simulink model "ECEN_5738_Project_sim"  (R2025b)
settings: Solver=VariableStepAuto  StartTime=0.0  StopTime=3  RelTol=1e-3
undefined symbols (not defined in the file): L, m, p1, p2, p3, p4, p5, r, v, x0
settings Model: Creator=jacks  LastModifiedBy=phil

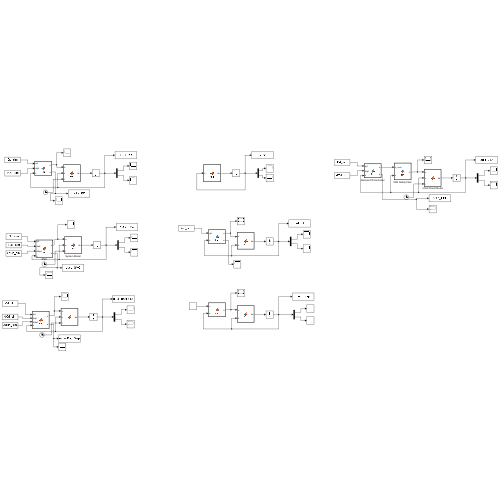
[thumbnail: Simulink's stored preview of the top-level diagram]
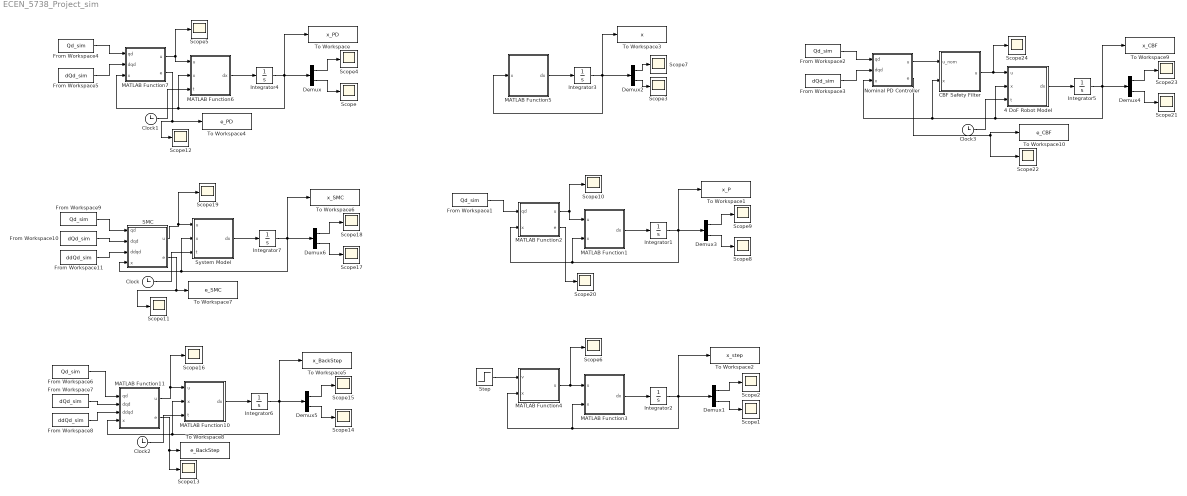
== system ECEN_5738_Project_sim ==
  4 DoF Robot Model : MATLAB Function  TreatAsAtomicUnit=on
  CBF Safety Filter : MATLAB Function  TreatAsAtomicUnit=on
  Clock{,1..3} (4 alike) : Clock
  Demux{,1..6} (7 alike) : Demux  Outputs=2
  From Workspace{1..2,4,6,9} (5 alike) : FromWorkspace  VariableName=Qd_sim
  From Workspace{3,5,7,10} (4 alike) : FromWorkspace  VariableName=dQd_sim
  From Workspace11 : FromWorkspace  VariableName=ddQd_sim
  From Workspace8 : FromWorkspace  VariableName=ddQd_sim
  Integrator{1..7} (7 alike) : Integrator  InitialCondition=x0
  MATLAB Function1 : MATLAB Function  TreatAsAtomicUnit=on
  MATLAB Function10 : MATLAB Function  TreatAsAtomicUnit=on
  MATLAB Function11 : MATLAB Function  TreatAsAtomicUnit=on
  MATLAB Function2 : MATLAB Function  TreatAsAtomicUnit=on
  MATLAB Function3 : MATLAB Function  TreatAsAtomicUnit=on
  MATLAB Function4 : MATLAB Function  TreatAsAtomicUnit=on
  MATLAB Function5 : MATLAB Function  TreatAsAtomicUnit=on
  MATLAB Function6 : MATLAB Function  TreatAsAtomicUnit=on
  MATLAB Function7 : MATLAB Function  TreatAsAtomicUnit=on
  Nominal PD Controller : MATLAB Function  TreatAsAtomicUnit=on
  SMC : MATLAB Function  TreatAsAtomicUnit=on
  Scope{,1..24} (25 alike) : Scope
      Scope settings: ActiveDisplayYMinimum=-1.04346  ActiveDisplayYMaximum=6.65946  DataLoggingVariableName=ScopeData3
      Scope1 settings: ActiveDisplayYMinimum=-0.94669  ActiveDisplayYMaximum=4.37778  DataLoggingVariableName=ScopeData4
      Scope10 settings: ActiveDisplayYMinimum=-1.20532  ActiveDisplayYMaximum=5.7236  DataLoggingVariableName=ScopeData8
      Scope11 settings: ActiveDisplayYMinimum=-0.00123  ActiveDisplayYMaximum=0.00133  DataLoggingVariableName=ScopeData4
      Scope12 settings: ActiveDisplayYMinimum=-0.0028  ActiveDisplayYMaximum=0.00283  DataLoggingVariableName=ScopeData5
      Scope13 settings: ActiveDisplayYMinimum=-0.01077  ActiveDisplayYMaximum=0.01072  DataLoggingVariableName=ScopeData6
      Scope14 settings: ActiveDisplayYMinimum=-1.05117  ActiveDisplayYMaximum=6.70832  DataLoggingVariableName=ScopeData14
      Scope15 settings: ActiveDisplayYMinimum=-2.41084  ActiveDisplayYMaximum=7.25873  DataLoggingVariableName=ScopeData15
      Scope16 settings: ActiveDisplayYMinimum=-4.58136  ActiveDisplayYMaximum=9.58212  DataLoggingVariableName=ScopeData16
      Scope17 settings: ActiveDisplayYMinimum=-1.0429937970844376  ActiveDisplayYMaximum=6.665414521803287
      Scope18 settings: ActiveDisplayYMinimum=-2.4103155124247957  ActiveDisplayYMaximum=7.2502189725166577  DataLoggingVariableName=ScopeData2
      Scope19 settings: ActiveDisplayYMinimum=-4.55981  ActiveDisplayYMaximum=9.43347  DataLoggingVariableName=ScopeData3
      Scope2 settings: ActiveDisplayYMinimum=-2.27232  ActiveDisplayYMaximum=6.12142
      Scope20 settings: ActiveDisplayYMinimum=-0.02858  ActiveDisplayYMaximum=0.02832  DataLoggingVariableName=ScopeData7
      Scope21 settings: ActiveDisplayYMinimum=-0.93914626541497248  ActiveDisplayYMaximum=5.7206527652501826
      Scope22 settings: ActiveDisplayYMinimum=-0.1369  ActiveDisplayYMaximum=0.37912  DataLoggingVariableName=ScopeData2
      Scope23 settings: ActiveDisplayYMinimum=-2.3974052419553082  ActiveDisplayYMaximum=7.1319937805003715  DataLoggingVariableName=ScopeData3
      Scope24 settings: ActiveDisplayYMinimum=-4.5558  ActiveDisplayYMaximum=9.43326  DataLoggingVariableName=ScopeData4
      Scope3 settings: ActiveDisplayYMinimum=-16.16611  ActiveDisplayYMaximum=1.79624
      Scope4 settings: ActiveDisplayYMinimum=-2.41035  ActiveDisplayYMaximum=7.2485  DataLoggingVariableName=ScopeData2
      Scope5 settings: ActiveDisplayYMinimum=-4.55909  ActiveDisplayYMaximum=9.43362  DataLoggingVariableName=ScopeData5
      Scope6 settings: ActiveDisplayYMinimum=-0.16415  ActiveDisplayYMaximum=1.38114  DataLoggingVariableName=ScopeData6
      Scope7 settings: ActiveDisplayYMinimum=-7.05771  ActiveDisplayYMaximum=2.87087  DataLoggingVariableName=ScopeData7
      Scope8 settings: ActiveDisplayYMinimum=-18.16231  ActiveDisplayYMaximum=18.17247  DataLoggingVariableName=ScopeData9
      Scope9 settings: ActiveDisplayYMinimum=-2.41317  ActiveDisplayYMaximum=7.27485  DataLoggingVariableName=ScopeData10
  Step : Step  Time=0  Before=x0(1:4)  After=v  SampleTime=0
  System Model : MATLAB Function  TreatAsAtomicUnit=on
  To Workspace : ToWorkspace  VariableName=x_PD  SaveFormat=Timeseries  SampleTime=-1
  To Workspace1 : ToWorkspace  VariableName=x_P  SaveFormat=Timeseries  SampleTime=-1
  To Workspace10 : ToWorkspace  VariableName=e_CBF  SaveFormat=Timeseries  SampleTime=-1
  To Workspace2 : ToWorkspace  VariableName=x_step  SaveFormat=Timeseries  SampleTime=-1
  To Workspace3 : ToWorkspace  VariableName=x  SaveFormat=Timeseries  SampleTime=-1
  To Workspace4 : ToWorkspace  VariableName=e_PD  SaveFormat=Timeseries  SampleTime=-1
  To Workspace5 : ToWorkspace  VariableName=x_BackStep  SaveFormat=Timeseries  SampleTime=-1
  To Workspace6 : ToWorkspace  VariableName=x_SMC  SaveFormat=Timeseries  SampleTime=-1
  To Workspace7 : ToWorkspace  VariableName=e_SMC  SaveFormat=Timeseries  SampleTime=-1
  To Workspace8 : ToWorkspace  VariableName=e_BackStep  SaveFormat=Timeseries  SampleTime=-1
  To Workspace9 : ToWorkspace  VariableName=x_CBF  SaveFormat=Timeseries  SampleTime=-1
  wires:
  Integrator2/1 -> To Workspace2/1, Demux1/1, MATLAB Function3/2(x), MATLAB Function4/2(x)
  MATLAB Function4/1(u) -> Scope6/1, MATLAB Function3/1(u)
  MATLAB Function3/1(dx) -> Integrator2/1
  Step/1 -> MATLAB Function4/1(v)
  Integrator3/1 -> To Workspace3/1, MATLAB Function5/1(x), Demux2/1
  MATLAB Function5/1(dx) -> Integrator3/1
  From Workspace5/1 -> MATLAB Function7/2(dqd)
  Integrator4/1 -> To Workspace/1, Demux/1, MATLAB Function7/3(x), MATLAB Function6/2(x)
  MATLAB Function6/1(dx) -> Integrator4/1
  MATLAB Function7/1(u) -> MATLAB Function6/1(u), Scope5/1
  From Workspace4/1 -> MATLAB Function7/1(qd)
  Demux/1 -> Scope4/1
  Demux/2 -> Scope/1
  Demux1/2 -> Scope1/1
  Demux1/1 -> Scope2/1
  Demux2/2 -> Scope3/1
  Demux2/1 -> Scope7/1
  Integrator1/1 -> To Workspace1/1, Demux3/1, MATLAB Function2/2(x), MATLAB Function1/2(x)
  MATLAB Function2/1(u) -> MATLAB Function1/1(u), Scope10/1
  From Workspace1/1 -> MATLAB Function2/1(qd)
  MATLAB Function1/1(dx) -> Integrator1/1
  Demux3/1 -> Scope9/1
  Demux3/2 -> Scope8/1
  Integrator6/1 -> To Workspace5/1, Demux5/1, MATLAB Function11/4(x), MATLAB Function10/2(x)
  From Workspace7/1 -> MATLAB Function11/2(dqd)
  MATLAB Function11/1(u) -> Scope16/1, MATLAB Function10/1(u)
  From Workspace6/1 -> MATLAB Function11/1(qd)
  MATLAB Function10/1(dx) -> Integrator6/1
  Demux5/1 -> Scope15/1
  Demux5/2 -> Scope14/1
  From Workspace8/1 -> MATLAB Function11/3(ddqd)
  From Workspace9/1 -> SMC/1(qd)
  Integrator7/1 -> To Workspace6/1, Demux6/1, SMC/4(x), System Model/2(x)
  From Workspace10/1 -> SMC/2(dqd)
  Demux6/2 -> Scope17/1
  System Model/1(dx) -> Integrator7/1
  Demux6/1 -> Scope18/1
  From Workspace11/1 -> SMC/3(ddqd)
  SMC/1(u) -> Scope19/1, System Model/1(u)
  Clock/1 -> System Model/3(t)
  Clock1/1 -> MATLAB Function6/3(t)
  Clock2/1 -> MATLAB Function10/3(t)
  MATLAB Function7/2(e) -> To Workspace4/1, Scope12/1
  SMC/2(e) -> Scope11/1, To Workspace7/1
  MATLAB Function11/2(e) -> Scope13/1, To Workspace8/1
  MATLAB Function2/2(e) -> Scope20/1
  4 DoF Robot Model/1(dx) -> Integrator5/1
  Demux4/1 -> Scope23/1
  Clock3/1 -> 4 DoF Robot Model/3(t)
  Demux4/2 -> Scope21/1
  Nominal PD Controller/2(e) -> To Workspace10/1, Scope22/1
  From Workspace2/1 -> Nominal PD Controller/1(qd)
  From Workspace3/1 -> Nominal PD Controller/2(dqd)
  Integrator5/1 -> To Workspace9/1, Demux4/1, CBF Safety Filter/2(x), Nominal PD Controller/3(x), 4 DoF Robot Model/2(x)
  Nominal PD Controller/1(u) -> CBF Safety Filter/1(u_nom)
  CBF Safety Filter/1(u) -> Scope24/1, 4 DoF Robot Model/1(u)

== matlab function ECEN_5738_Project_sim/MATLAB Function7 ==
  data: qd input; dqd input; x input; u output; e output
function [u,e] =  fcn(qd, dqd, x)


kp = [1500; 2500; 1250; 750];
kd = [1050; 1750; 875; 1225];

q  = [x(1); x(2); x(3); x(4)];
dq = [x(5); x(6); x(7); x(8)];

e  = qd - q;
de = dqd - dq;

u = kp.*e + kd.*de;
end

== matlab function ECEN_5738_Project_sim/4 DoF Robot Model ==
  data: u input; x input; t input; dx output; L parameter; m parameter; r parameter; p1 parameter; p2 parameter; p3 parameter; p4 parameter; p5 parameter
function dx = fcn(u, x, t, L, m, r, p1, p2, p3, p4, p5)

q  = [x(1); x(2); x(3); x(4)];  %theta
dq = [x(5); x(6); x(7); x(8)];  %theta-dot

p6 = (L(3)*m(3)+L(3)*m(4)+m(3)*r(3))*L(1)*sin(q(3));

M = [p1+p2*cos(q(3))     0   p3+0.5*p2*cos(q(3))  p5
            0            p4            0          0
     p3+0.5*p2*cos(q(3)) 0             p3         p5
            p5           0             p5         p5];

C = [-dq(3)          0     -(dq(1)+dq(3))*p6      0
         0           0              0             0
     dq(1)*p6        0              0             0
         0           0              0             0];

G = [0; 9.81*(m(2)+m(3)+m(4)); 0; 0];

omega = 5;
D0 = 3*cos(omega*t) + 0.5*sin(omega*t);

D = [D0; D0; D0; 0];


dx = [dq; M \ (u-C*dq-G-D)];



end

== matlab function ECEN_5738_Project_sim/Nominal PD Controller ==
  data: qd input; dqd input; x input; u output; e output
function [u,e] =  fcn(qd, dqd, x)


kp = [1500; 2500; 1250; 750];
kd = [1050; 1750; 875; 1225];

q  = [x(1); x(2); x(3); x(4)];
dq = [x(5); x(6); x(7); x(8)];

e  = qd - q;
de = dqd - dq;

u = kp.*e + kd.*de;
end

== matlab function ECEN_5738_Project_sim/MATLAB Function10 ==
  data: u input; x input; t input; dx output; L parameter; m parameter; r parameter; p1 parameter; p2 parameter; p3 parameter; p4 parameter; p5 parameter
function dx = fcn(u, x, t, L, m, r, p1, p2, p3, p4, p5)

q  = [x(1); x(2); x(3); x(4)];  %theta
dq = [x(5); x(6); x(7); x(8)];  %theta-dot

p6 = (L(3)*m(3)+L(3)*m(4)+m(3)*r(3))*L(1)*sin(q(3));

M = [p1+p2*cos(q(3))     0   p3+0.5*p2*cos(q(3))  p5
            0            p4            0          0
     p3+0.5*p2*cos(q(3)) 0             p3         p5
            p5           0             p5         p5];

C = [-dq(3)          0     -(dq(1)+dq(3))*p6      0
         0           0              0             0
     dq(1)*p6        0              0             0
         0           0              0             0];

G = [0; 9.81*(m(2)+m(3)+m(4)); 0; 0];

omega = 5;
D0 = 3*cos(omega*t) + 0.5*sin(omega*t);

D = [D0; D0; D0; 0];

dx = [dq; M \ (u-C*dq-G-D)];



end

== matlab function ECEN_5738_Project_sim/MATLAB Function11 ==
  data: qd input; dqd input; ddqd input; x input; u output; r parameter; m parameter; L parameter; p5 parameter; p4 parameter; p3 parameter; p2 parameter; p1 parameter; e output
function [u,e] = fcn(qd, dqd, ddqd, x, r, m, L, p5, p4, p3, p2, p1)

q  = x(1:4);
dq = x(5:8);

p6 = (L(3)*m(3)+L(3)*m(4)+m(3)*r(3))*L(1)*sin(q(3));

M = [p1+p2*cos(q(3))      0   p3+0.5*p2*cos(q(3))   p5
            0             p4           0            0
     p3+0.5*p2*cos(q(3))  0            p3           p5
            p5            0            p5           p5];

C = [ -dq(3)          0     -(dq(1)+dq(3))*p6    0
          0           0              0           0
      dq(1)*p6        0              0           0
          0           0              0           0 ];

G = [0;9.81*(m(2)+m(3)+m(4));0;0];

% Backstepping gains
K1 = diag([50 50 50 50]);
K2 = diag([300 300 280 280]);

% position error
e1 = q - qd;

% Virtual control
alpha = dqd - K1*e1;

% velocity error
e2 = dq - alpha;

% alpha dot
alpha_dot = ddqd - K1*(dq - dqd);

% Backstepping control
tau = M*(alpha_dot - K2*e2 - e1) + C*dq + G;

u = tau;

e = e1;
end

== matlab function ECEN_5738_Project_sim/System Model ==
  data: u input; x input; t input; dx output; L parameter; m parameter; r parameter; p1 parameter; p2 parameter; p3 parameter; p4 parameter; p5 parameter
function dx = fcn(u, x, t, L, m, r, p1, p2, p3, p4, p5)

q  = [x(1); x(2); x(3); x(4)];  %theta
dq = [x(5); x(6); x(7); x(8)];  %theta-dot

p6 = (L(3)*m(3)+L(3)*m(4)+m(3)*r(3))*L(1)*sin(q(3));

M = [p1+p2*cos(q(3))     0   p3+0.5*p2*cos(q(3))  p5
            0            p4            0          0
     p3+0.5*p2*cos(q(3)) 0             p3         p5
            p5           0             p5         p5];

C = [-dq(3)          0     -(dq(1)+dq(3))*p6      0
         0           0              0             0
     dq(1)*p6        0              0             0
         0           0              0             0];

G = [0; 9.81*(m(2)+m(3)+m(4)); 0; 0];

omega = 5;
D0 = 3*cos(omega*t) + 0.5*sin(omega*t);

D = [D0; D0; D0; 0];

dx = [dq; M \ (u-C*dq-G-D)];


end

== matlab function ECEN_5738_Project_sim/SMC ==
  data: qd input; dqd input; ddqd input; x input; u output; r parameter; m parameter; L parameter; p5 parameter; p4 parameter; p3 parameter; p2 parameter; p1 parameter; e output
function [u,e] = fcn(qd, dqd, ddqd, x, r, m, L, p5, p4, p3, p2, p1)

q  = x(1:4);
dq = x(5:8);

p6 = (L(3)*m(3)+L(3)*m(4)+m(3)*r(3))*L(1)*sin(q(3));

M = [p1+p2*cos(q(3))      0   p3+0.5*p2*cos(q(3))   p5
            0             p4           0            0
     p3+0.5*p2*cos(q(3))  0            p3           p5
            p5            0            p5           p5];

C = [-dq(3)*p6       0   -(dq(1)+dq(3))*p6   0
          0          0            0          0
      dq(1)*p6       0            0          0
          0          0            0          0];

G = [0; 9.81*(m(2)+m(3)+m(4)); 0; 0];

e  = qd - q;
de = dqd - dq;

Lambda = diag([20 20 20 20]);
K      = diag([400 400 300 300]);

s = de + Lambda*e;

phi = 0.05;
sat_s = min(abs(s/phi),1).*sign(s);
v = ddqd + Lambda*de + K*sat_s;

tau = M*v + C*dq + G;

u = tau;
end

== matlab function ECEN_5738_Project_sim/CBF Safety Filter ==
  data: u_nom input; x input; u output
function u = fcn(u_nom, x)
%#codegen
coder.extrinsic('quadprog')
coder.extrinsic('optimoptions')


alpha = 5000;

A = [-Lg_h1_fun(x)
     -Lg_h2_fun(x)
     -Lg_h3_fun(x)
     -Lg_h4_fun(x)];

b = [Lf_h1_fun(x) + alpha*h1_fun(x)
     Lf_h2_fun(x) + alpha*h2_fun(x)
     Lf_h3_fun(x) + alpha*h3_fun(x)
     Lf_h4_fun(x) + alpha*h4_fun(x)];

u = zeros(4,1);

u = quadprog(eye(4),-u_nom,A,b,[],[],[],[],[],optimoptions('quadprog','Display','none'));


end

== matlab function ECEN_5738_Project_sim/MATLAB Function1 ==
  data: u input; x input; dx output; L parameter; m parameter; r parameter; p1 parameter; p2 parameter; p3 parameter; p4 parameter; p5 parameter
function dx = fcn(u, x, L, m, r, p1, p2, p3, p4, p5)

q  = [x(1); x(2); x(3); x(4)];  %theta
dq = [x(5); x(6); x(7); x(8)];  %theta-dot

p6 = (L(3)*m(3)+L(3)*m(4)+m(3)*r(3))*L(1)*sin(q(3));

M = [p1+p2*cos(q(3))     0   p3+0.5*p2*cos(q(3))  p5
            0            p4            0          0
     p3+0.5*p2*cos(q(3)) 0             p3         p5
            p5           0             p5         p5];

C = [-dq(3)          0     -(dq(1)+dq(3))*p6      0
         0           0              0             0
     dq(1)*p6        0              0             0
         0           0              0             0];

G = [0; 9.81*(m(2)+m(3)+m(4)); 0; 0];

dx = [dq; M \ (u-C*dq-G)];


end

== matlab function ECEN_5738_Project_sim/MATLAB Function3 ==
  data: u input; x input; dx output; L parameter; m parameter; r parameter; p1 parameter; p2 parameter; p3 parameter; p4 parameter; p5 parameter
function dx = fcn(u, x, L, m, r, p1, p2, p3, p4, p5)

q  = [x(1); x(2); x(3); x(4)];  %theta
dq = [x(5); x(6); x(7); x(8)];  %theta-dot

p6 = (L(3)*m(3)+L(3)*m(4)+m(3)*r(3))*L(1)*sin(q(3));

M = [p1+p2*cos(q(3))     0   p3+0.5*p2*cos(q(3))  p5
            0            p4            0          0
     p3+0.5*p2*cos(q(3)) 0             p3         p5
            p5           0             p5         p5];

C = [-dq(3)          0     -(dq(1)+dq(3))*p6      0
         0           0              0             0
     dq(1)*p6        0              0             0
         0           0              0             0];

G = [0; 9.81*(m(2)+m(3)+m(4)); 0; 0];

dx = [dq; M \ (u-C*dq-G.*q)];


end

== matlab function ECEN_5738_Project_sim/MATLAB Function2 ==
  data: qd input; x input; u output; e output
function [u,e] =  fcn(qd, x)


kp = [1500; 2500; 1250; 750];

q  = [x(1); x(2); x(3); x(4)];

e  = qd - q;

u = kp.*e;
end

== matlab function ECEN_5738_Project_sim/MATLAB Function4 ==
  data: v input; x input; u output
function u =  fcn(v, x)


kp = [1500; 2500; 1250; 750];
kd = [1050; 1750; 875; 1225];

q  = [x(1); x(2); x(3); x(4)];
dq = [x(5); x(6); x(7); x(8)];

e  = v - q;
de =  - dq;

u = kp.*e + kd.*de;
end

== matlab function ECEN_5738_Project_sim/MATLAB Function5 ==
  data: x input; dx output; L parameter; m parameter; r parameter; p1 parameter; p2 parameter; p3 parameter; p4 parameter; p5 parameter
function dx = fcn(x, L, m, r, p1, p2, p3, p4, p5)

q  = [x(1); x(2); x(3); x(4)];  %theta
dq = [x(5); x(6); x(7); x(8)];  %theta-dot

p6 = (L(3)*m(3)+L(3)*m(4)+m(3)*r(3))*L(1)*sin(q(3));

M = [p1+p2*cos(q(3))     0   p3+0.5*p2*cos(q(3))  p5
            0            p4            0          0
     p3+0.5*p2*cos(q(3)) 0             p3         p5
            p5           0             p5         p5];

C = [-dq(3)          0     -(dq(1)+dq(3))*p6      0
         0           0              0             0
     dq(1)*p6        0              0             0
         0           0              0             0];

G = [0; 9.81*(m(2)+m(3)+m(4)); 0; 0];

dx = [dq; M \ (-C*dq-G)];


end

== matlab function ECEN_5738_Project_sim/MATLAB Function6 ==
  data: u input; x input; t input; dx output; L parameter; m parameter; r parameter; p1 parameter; p2 parameter; p3 parameter; p4 parameter; p5 parameter
function dx = fcn(u, x, t, L, m, r, p1, p2, p3, p4, p5)

q  = [x(1); x(2); x(3); x(4)];  %theta
dq = [x(5); x(6); x(7); x(8)];  %theta-dot

p6 = (L(3)*m(3)+L(3)*m(4)+m(3)*r(3))*L(1)*sin(q(3));

M = [p1+p2*cos(q(3))     0   p3+0.5*p2*cos(q(3))  p5
            0            p4            0          0
     p3+0.5*p2*cos(q(3)) 0             p3         p5
            p5           0             p5         p5];

C = [-dq(3)          0     -(dq(1)+dq(3))*p6      0
         0           0              0             0
     dq(1)*p6        0              0             0
         0           0              0             0];

G = [0; 9.81*(m(2)+m(3)+m(4)); 0; 0];

omega = 5;
D0 = 3*cos(omega*t) + 0.5*sin(omega*t);

D = [D0; D0; D0; 0];


dx = [dq; M \ (u-C*dq-G-D)];



end
